simulink model "linear_system"  (R2024a)
settings: Solver=VariableStepAuto  StartTime=0.0  StopTime=60  RelTol=1e-3
settings Model: Creator=alexandr  LastModifiedBy=alexandr

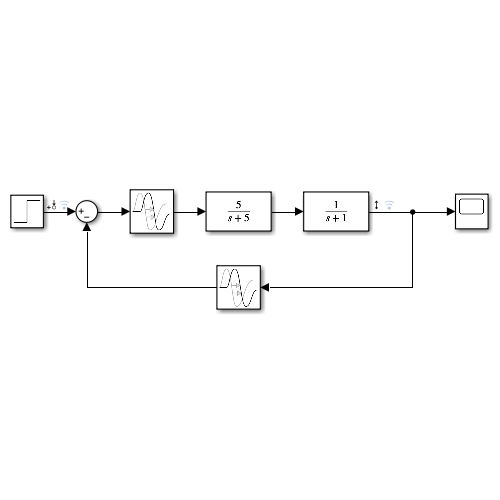
[thumbnail: Simulink's stored preview of the top-level diagram]
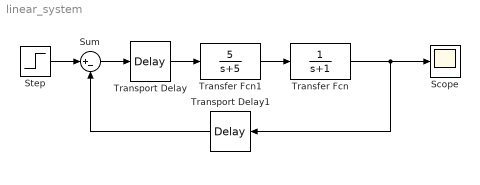
== system linear_system ==
  Scope : Scope
  Step : Step  SampleTime=0
  Sum : Sum  Inputs=|+-
  Transfer Fcn : TransferFcn  Denominator=[1 1]
  Transfer Fcn1 : TransferFcn  Numerator=[5]  Denominator=[1 5]
  Transport Delay : TransportDelay
  Transport Delay1 : TransportDelay
  wires:
  Sum/1 -> Transport Delay/1
  Transport Delay/1 -> Transfer Fcn1/1
  Transfer Fcn1/1 -> Transfer Fcn/1
  Transfer Fcn/1 -> Transport Delay1/1, Scope/1
  Transport Delay1/1 -> Sum/2
  Step/1 -> Sum/1
